simulink model "simulink_model"  (R2024b)
settings: Solver=VariableStepAuto  StartTime=0.0  StopTime=1  RelTol=1e-3
undefined symbols (not defined in the file): jsin
libraries: commsdrhw_v2 x2
settings Model: Creator=MEDHA TRUST  LastModifiedBy=MEDHA TRUST
settings OptimizationCC: ReuseModelBlockBuffer=off
settings RTWCC: GPUComputeCapability=3.5

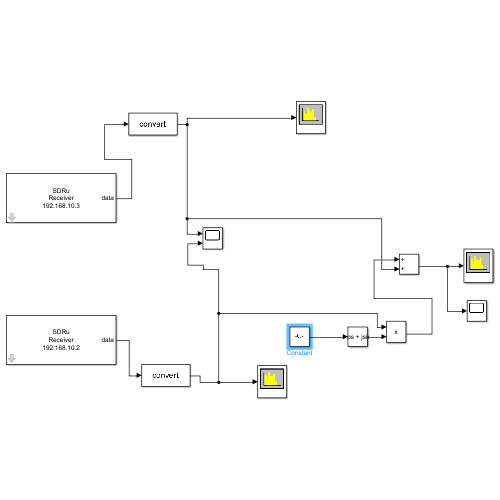
[thumbnail: Simulink's stored preview of the top-level diagram]
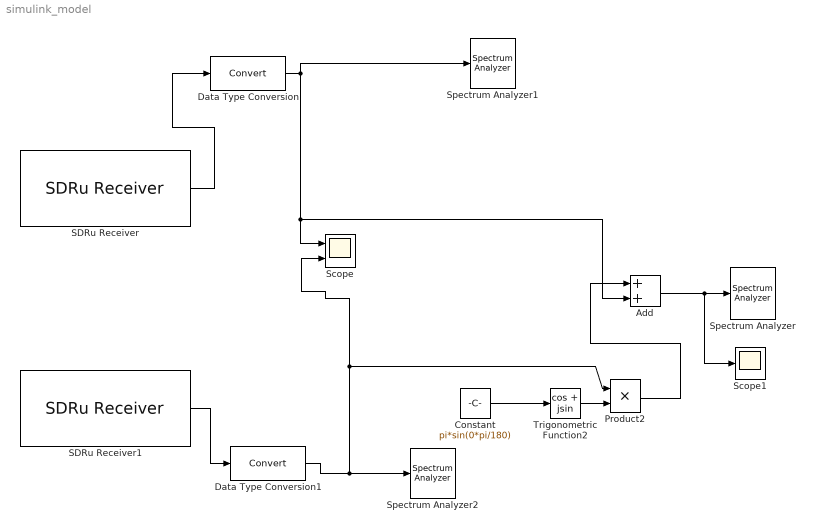
== system simulink_model ==
  Add : Sum
  Constant : Constant  Value=pi*sin(0*pi/180)
  Data Type Conversion : DataTypeConversion  SaturateOnIntegerOverflow=off  RndMeth=Floor
  Data Type Conversion1 : DataTypeConversion  SaturateOnIntegerOverflow=off  RndMeth=Floor
  Product2 : Product
  SDRu Receiver : commsdrhw_v2/SDRu Receiver  rxtx=rx  initializeIPAddress=0  devMap=10  USRP2_IP=192.168.10.3  USRP_IP_X300=192.168.10.2  USRP_IP_X310=No devices found  USRP_IP_N300=192.168.10.2  USRP_IP_N310=192.168.10.2  USRP_IP_N320=192.168.10.2  USRP_serialNumB200=No devices found  USRP_serialNumB210=3136D21  platform=N200/N210/USRP2  prevPlatform=N200/N210/USRP2  lastIPAddressPopup=192.168.10.2  USRP_ID=192.168.10.3  LastIPAddress=192.168.10.2  IsTwinRXDaughterboard=off  EnableTwinRXPhaseSync=off  losrc=0  ChannelMapping=1  centerFrequencySrc=Dialog  centerFrequency=2.3e9  loOffsetSrc=Dialog  loOffset=0  gainSrc=Dialog  gain=1  PPSSource=External  clockSource=External  EnableGPSLock=off  EnsureSyncGPSTime=off  EnableTimeTrigger=off  triggerTime=5  enableMIMOCableSync=off  EnableRefLock=off  masterClkRateParam=100e6  masterClkRateB200=32e6  masterClkRateB210=32e6  masterClkRateX300=200e6  masterClkRateX310=200e6  masterClkRateN300=125e6  masterClkRateN310=125e6  masterClkRateN320=200e6  masterClkRate=100e6  masterClkRateTwinRX=200e6  decimInterpSrc=Dialog  decimInterpPort=512  lastDecimSource=Dialog  decimInterp=120  USRP2_IP_NUM=[49 57 50 46 49 54 56 46 49 48 46 51]  sampleRate=833333.33333333337  sampleTime=(120)/100000000  TransportDataType=int16  overrunUnderrunPort=off  dataLengthPort=off  EnableTimeStamps=off  outputDatatype=Same as transport data type  frameLength=1  HOST_DATA_PORT=0  HOST_CONTROL_PORT=0  USRP2_DATA_PORT=0  USRP2_CONTROL_PORT=0  bufferMode=Continuous streaming  EnableBurstMode=off  NumFramesInBurst=100
  SDRu Receiver1 : commsdrhw_v2/SDRu Receiver  rxtx=rx  initializeIPAddress=0  devMap=10  USRP2_IP=192.168.10.2  USRP_IP_X300=192.168.10.2  USRP_IP_X310=No devices found  USRP_IP_N300=192.168.10.2  USRP_IP_N310=192.168.10.2  USRP_IP_N320=192.168.10.2  USRP_serialNumB200=No devices found  USRP_serialNumB210=3136D21  platform=N200/N210/USRP2  prevPlatform=N200/N210/USRP2  lastIPAddressPopup=192.168.10.2  USRP_ID=192.168.10.2  LastIPAddress=192.168.10.2  IsTwinRXDaughterboard=off  EnableTwinRXPhaseSync=off  losrc=0  ChannelMapping=1  centerFrequencySrc=Dialog  centerFrequency=2.3e9  loOffsetSrc=Dialog  loOffset=0  gainSrc=Dialog  gain=25  PPSSource=External  clockSource=External  EnableGPSLock=off  EnsureSyncGPSTime=off  EnableTimeTrigger=off  triggerTime=5  enableMIMOCableSync=off  EnableRefLock=off  masterClkRateParam=100e6  masterClkRateB200=32e6  masterClkRateB210=32e6  masterClkRateX300=200e6  masterClkRateX310=200e6  masterClkRateN300=125e6  masterClkRateN310=125e6  masterClkRateN320=200e6  masterClkRate=100e6  masterClkRateTwinRX=200e6  decimInterpSrc=Dialog  decimInterpPort=512  lastDecimSource=Dialog  decimInterp=120  USRP2_IP_NUM=[49 57 50 46 49 54 56 46 49 48 46 50]  sampleRate=833333.33333333337  sampleTime=(120)/100000000  TransportDataType=int16  overrunUnderrunPort=off  dataLengthPort=off  EnableTimeStamps=off  outputDatatype=Same as transport data type  frameLength=1  HOST_DATA_PORT=0  HOST_CONTROL_PORT=0  USRP2_DATA_PORT=0  USRP2_CONTROL_PORT=0  bufferMode=Continuous streaming  EnableBurstMode=off  NumFramesInBurst=100
  Scope : Scope  NumInputPorts=2
  Scope1 : Scope
  Spectrum Analyzer : SpectrumAnalyzer  WindowPosition=[642.000000,362.000000,637.000000,328.000000,]  Visible=on  ScopeFrameLocation=window  SampleRate=833333.333333333  Span=833333.333333333  StartFrequency=-416666.666666667  StopFrequency=416666.666666667  AveragingMethod=Exponential  YLimits=[-3.41699277,110.62551052]  AllowFFTLengthLessThanSamplesPerUpdate=on
  Spectrum Analyzer1 : SpectrumAnalyzer  WindowPosition=[2.000000,362.000000,637.000000,328.000000,]  Visible=on  ScopeFrameLocation=window  WindowInvariantSamplesPerUpdate=on  Span=833333.3333333334  StartFrequency=-416666.6666666667  StopFrequency=416666.6666666667  YLimits=[-8.77105725,102.51437118]  SelectedToolstripTab=spectrumAnalyzerToolstrip.measurementsTab
  Spectrum Analyzer2 : SpectrumAnalyzer  WindowPosition=[2.000000,2.000000,637.000000,328.000000,]  Visible=on  ScopeFrameLocation=window  WindowInvariantSamplesPerUpdate=on  Span=833333.3333333334  StartFrequency=-416666.6666666667  StopFrequency=416666.6666666667  YLimits=[-4.68453986,106.25614868]  SelectedToolstripTab=spectrumAnalyzerToolstrip.measurementsTab
  Trigonometric Function2 : Trigonometry  Operator=cos + jsin
  wires:
  SDRu Receiver/1 -> Data Type Conversion/1
  Data Type Conversion/1 -> Spectrum Analyzer1/1, Add/2, Scope/1
  SDRu Receiver1/1 -> Data Type Conversion1/1
  Data Type Conversion1/1 -> Spectrum Analyzer2/1, Scope/2, Product2/1
  Add/1 -> Scope1/1, Spectrum Analyzer/1
  Constant/1 -> Trigonometric Function2/1
  Trigonometric Function2/1 -> Product2/2
  Product2/1 -> Add/1
